simulink model "Motor_sim"  (R2018a)
settings: Solver=VariableStepAuto  StartTime=0.0  StopTime=10.0  RelTol=1e-3
values from neighbouring files (symbols this model uses):
  b = [0;1]    [Project_state_space.m]
  L = [l1; l2]    [Project_state_space.m]
undefined symbols (not defined in the file or in its folder): Jm, Ke, Kt, Ra
settings Model: Creator=Lenovo  LastModifiedBy=Lenovo

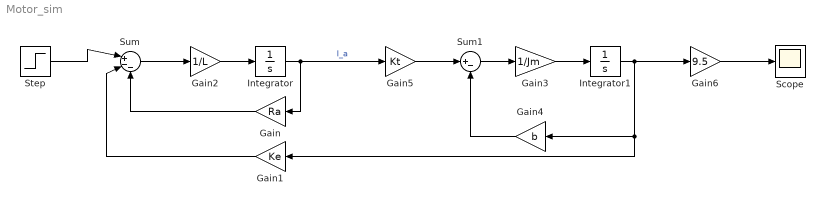
== system Motor_sim ==
  Gain : Gain  Gain=Ra
  Gain1 : Gain  Gain=Ke
  Gain2 : Gain  Gain=1/L
  Gain3 : Gain  Gain=1/Jm
  Gain4 : Gain  Gain=b
  Gain5 : Gain  Gain=Kt
  Gain6 : Gain  Gain=9.5
  Integrator : Integrator
  Integrator1 : Integrator
  Scope : Scope
  Step : Step  After=5  SampleTime=0
  Sum : Sum  Inputs=|+--
  Sum1 : Sum  Inputs=|+-
  wires:
  Integrator/1 -> Gain5/1, Gain/1  "I_a"
  Gain/1 -> Sum/3
  Gain1/1 -> Sum/2
  Step/1 -> Sum/1
  Sum/1 -> Gain2/1
  Gain2/1 -> Integrator/1
  Sum1/1 -> Gain3/1
  Gain3/1 -> Integrator1/1
  Integrator1/1 -> Gain6/1, Gain1/1, Gain4/1
  Gain4/1 -> Sum1/2
  Gain5/1 -> Sum1/1
  Gain6/1 -> Scope/1
